simulink model "Transformer"  (R2018b)
settings: Solver=VariableStepAuto  StartTime=0.0  StopTime=0.1  RelTol=1e-3
libraries: powerlib x17
settings Model: Creator=Vishant  LastModifiedBy=Vishant

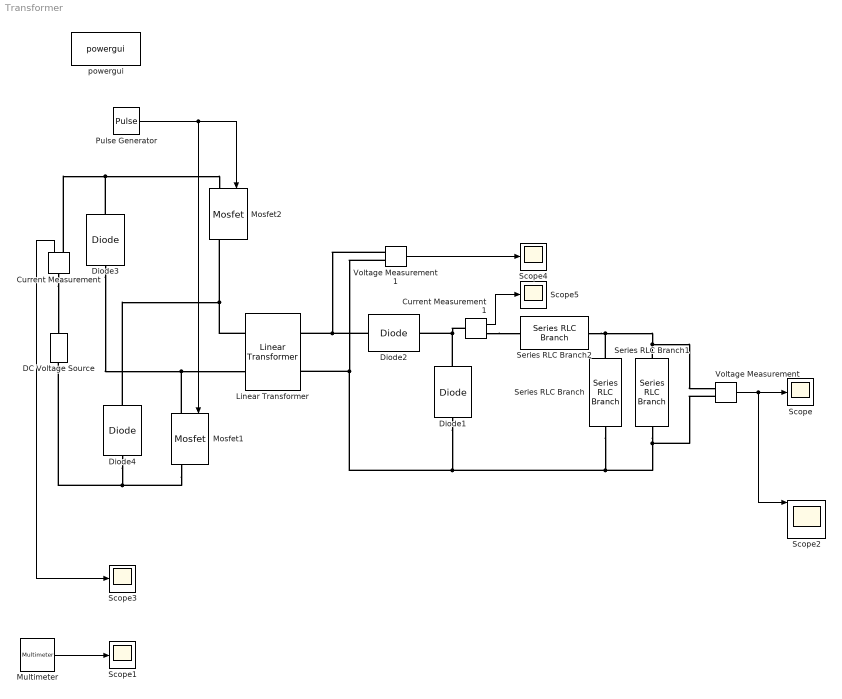
== system Transformer ==
  Current Measurement : powerlib/Measurements/Current Measurement  PhasorSimulation=off  OutputType=Complex  PSBequivalent=0
  Current Measurement1 : powerlib/Measurements/Current Measurement  PhasorSimulation=off  OutputType=Complex  PSBequivalent=0
  DC Voltage Source : powerlib/Electrical Sources/DC Voltage Source  Amplitude=330  Measurements=None
  Diode{1..4} (4 alike) : powerlib/Power Electronics/Diode  Ron=1e-10  Lon=0  Vf=0  IC=0  UseSnubber=0  Rs=inf  Cs=0  Measurements=off
  Linear Transformer : powerlib/Elements/Linear Transformer  UNITS=SI  NominalPower=[240 100e3]  winding1=[330 0 0]  winding2=[33 0 0]  ThreeWindings=off  winding3=[330 0 0]  RmLm=[inf 10e-3]  Measurements=All voltages and currents  DataType=on
  Mosfet1 : powerlib/Power Electronics/Mosfet  Ron=1e-10  Lon=0  Rd=1e-10  Vfd=1e-10  IC=0  Rs=1e5  Cs=0  Measurements=on
  Mosfet2 : powerlib/Power Electronics/Mosfet  Ron=1e-10  Lon=0  Rd=1e-10  Vfd=1e-10  IC=0  Rs=1e5  Cs=0  Measurements=on
  Multimeter : powerlib/Measurements/Multimeter  PhasorSimulation=off  OutputType=Complex  sel=6  L=7  Gain=1  yselected={'Imag: Linear Transformer'};  PSBOutputType=1  PSBequivalent=0  AxesSetting=[0,0.1,-100,100]  Display=0  SavedBlockNames=-11
  Pulse Generator : DiscretePulseGenerator  PulseType=Time based  Period=1/100000  PulseWidth=25.71
  Scope{,1,3..5} (5 alike) : Scope
  Scope2 : Scope  NumInputPorts=5
  Series RLC Branch : powerlib/Elements/Series RLC Branch  LConnTagsString=__new0  RConnTagsString=__new0  BranchType=C  Resistance=1  Inductance=1e-3  SetiL0=off  InitialCurrent=0  Capacitance=4.166e-6  Setx0=off  InitialVoltage=0  Measurements=None
  Series RLC Branch1 : powerlib/Elements/Series RLC Branch  LConnTagsString=__new0  RConnTagsString=__new0  BranchType=R  Resistance=6  Inductance=1e-3  SetiL0=off  InitialCurrent=0  Capacitance=1e-6  Setx0=off  InitialVoltage=0  Measurements=None
  Series RLC Branch2 : powerlib/Elements/Series RLC Branch  LConnTagsString=__new0  RConnTagsString=__new0  BranchType=L  Resistance=1  Inductance=12.83e-6  SetiL0=off  InitialCurrent=0  Capacitance=1e-6  Setx0=off  InitialVoltage=0  Measurements=None
  Voltage Measurement : powerlib/Measurements/Voltage Measurement  PhasorSimulation=off  OutputType=Complex  PSBequivalent=0
  Voltage Measurement1 : powerlib/Measurements/Voltage Measurement  PhasorSimulation=off  OutputType=Complex  PSBequivalent=0
  powergui : powerlib/powergui  Priority=1  SimulationMode=Continuous  SampleTime=0.000001  frequency=60  Iterations=50  frequencyindice=0  Pbase=100e6  ErrMax=1e-4  UnitsV=kV  UnitsW=MW  buscounter=0  FunctionMessages=off  echomessages=off  EnableUseOfTLC=off  CurrentSourceSwitches=off  DisableSnubberDevices=off  DisableRonSwitches=off  DisableVfSwitches=off  DisplayEquations=off  SolverType=Tustin/Backward Euler (TBE)  Interpol=off  ExternalGateDelay=off  methode=off  Ts=100  x0status=blocks  SPID=on  SwTol=0  HookPort=off  RestoreLinks=warning  ResistiveCurrentMeasurement=off  Frange=[0:2:500]  Ylog=off  Xlog=on  ShowGrid=off  save=off  variable=ZData  structure=0  ZoomFFT=off  StartTime=0.0  cycles=1  DisplayStyle=1  fundamental=60  FreqAxis=off  MaxFrequency=1000  frequencyindicesteady=1  RmsSteady=1  display=off
  wires:
  Pulse Generator/1 -> Mosfet2/1, Mosfet1/1
  Multimeter/1 -> Scope1/1
  Current Measurement/1 -> Scope3/1
  Voltage Measurement/1 -> Scope2/1, Scope/1
  Voltage Measurement1/1 -> Scope4/1
  Current Measurement1/1 -> Scope5/1
  connections:
  DC Voltage Source/LConn1 -- Mosfet1/RConn1 -- Diode4/LConn1
  Diode2/LConn1 -- Voltage Measurement1/LConn1 -- Linear Transformer/RConn1
  Diode1/RConn1 -- Current Measurement1/LConn1 -- Diode2/RConn1
  Voltage Measurement/LConn2 -- Diode1/LConn1 -- Voltage Measurement1/LConn2 -- Linear Transformer/RConn2 -- Series RLC Branch/RConn1 -- Series RLC Branch1/RConn1
  Mosfet1/LConn1 -- Diode3/LConn1 -- Linear Transformer/LConn2
  Diode4/RConn1 -- Linear Transformer/LConn1 -- Mosfet2/RConn1
  Diode3/RConn1 -- Current Measurement/RConn1 -- Mosfet2/LConn1
  Series RLC Branch1/LConn1 -- Series RLC Branch/LConn1 -- Series RLC Branch2/RConn1 -- Voltage Measurement/LConn1
  Current Measurement/LConn1 -- DC Voltage Source/RConn1
  Current Measurement1/RConn1 -- Series RLC Branch2/LConn1
